simulink library "netZeroSpoolingController_ul"  (R2018b)
settings: Solver=VariableStepAuto  StartTime=0.0  StopTime=10.0  RelTol=1e-3
undefined symbols (not defined in the file or in its folder): hiLvlCtrl
libraries: simulink x2, dspsigops x1, runningAvg_ul x1
settings Model: Creator=James Reed  LastModifiedBy=mcobb

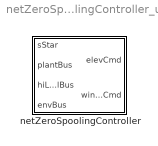
== system netZeroSpoolingController_ul ==
  netZeroSpoolingController : Subsystem  mask{L0=hiLvlCtrl.basisParams.Value(5), reelInDefl=23, reelOutDefl=0, sigmaVecInit=0}
      mask prompts: L0 "Target Tether Length"; reelInDefl "Reel In Elevator Deflection [deg]"; reelOutDefl "Reel Out Elevator Deflection [deg]"; sigmaVecInit "Init Spooling Param Vec [center width]"
      mask TypeOptions L0: TargetTetherLength/Value
      mask TypeOptions reelInDefl: ReelInElevDefl/Value
      mask TypeOptions reelOutDefl: ReelOutElevDefl/Value

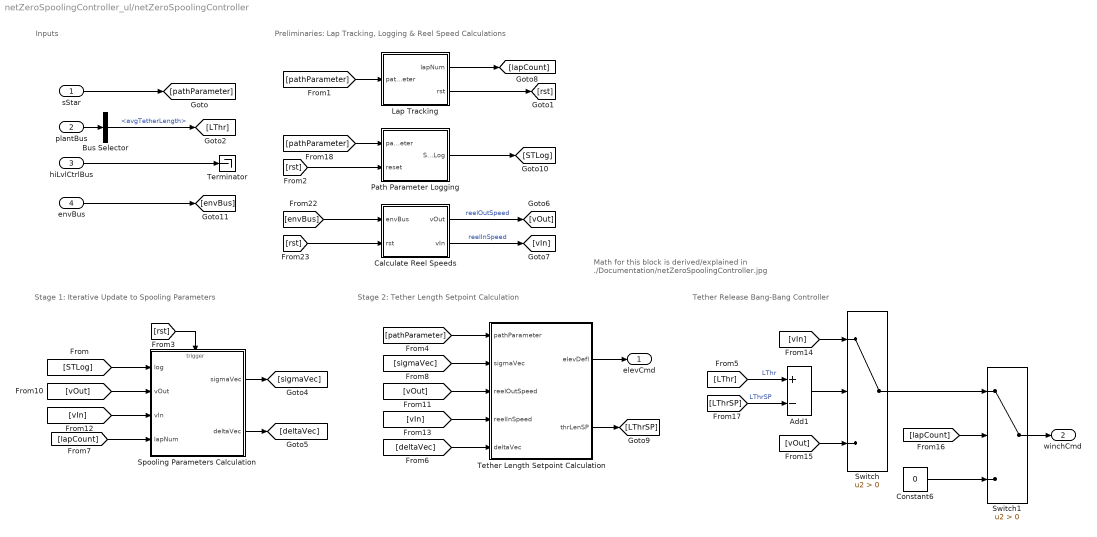
== system netZeroSpoolingController_ul/netZeroSpoolingController ==
  note: Math for this block is derived/explained in
      | ./Documentation/netZeroSpoolingController.jpg
  note: Stage 1: Iterative Update to Spooling Parameters
  note: Tether Release Bang-Bang Controller
  note: Stage 2: Tether Length Setpoint Calculation
  note: Inputs
  note: Preliminaries: Lap Tracking, Logging & Reel Speed Calculations
  "sStar " : Inport
  plantBus : Inport  Port=2  OutDataTypeStr=Bus: plantBus
  hiLvlCtrlBus : Inport  Port=3  OutDataTypeStr=Bus: hiLvlCtrlBus
  envBus : Inport  Port=4  OutDataTypeStr=Bus: envBus
  Add1 : Sum  Inputs=+-
  Bus Selector : BusSelector  OutputSignals=avgTetherLength
  Calculate Reel Speeds : Subsystem
  Constant6 : Constant  Value=0
  Lap Tracking : Subsystem
  Path Parameter Logging : Subsystem
  Spooling Parameters Calculation : Subsystem  TreatAsAtomicUnit=on
  Switch : Switch  Criteria=u2 > Threshold
  Switch1 : Switch  Criteria=u2 > Threshold
  Terminator : Terminator
  Tether Length Setpoint Calculation : Subsystem
  elevCmd : Outport
  "winchCmd " : Outport  Port=2
  wires:
  hiLvlCtrlBus/1 -> Terminator/1
  plantBus/1 -> Bus Selector/1
  "sStar "/1 -> [pathParameter]
  [rst] -> Spooling Parameters Calculation/Trigger
  Bus Selector/1 -> [LThr]  "<avgTetherLength>"
  [LThr] -> Add1/1  "LThr"
  Add1/1 -> Switch/2
  Spooling Parameters Calculation/1(sigmaVec) -> [sigmaVec]
  Spooling Parameters Calculation/2(deltaVec) -> [deltaVec]
  [vOut] -> Spooling Parameters Calculation/2(vOut)
  [vIn] -> Spooling Parameters Calculation/3(vIn)
  Switch1/1 -> "winchCmd "/1
  [LThrSP] -> Add1/2  "LThrSP"
  [vIn] -> Switch/1
  [vOut] -> Switch/3
  [lapCount] -> Switch1/2
  Switch/1 -> Switch1/1
  Constant6/1 -> Switch1/3
  [pathParameter] -> Path Parameter Logging/1(pathParameter)
  [rst] -> Path Parameter Logging/2(reset)
  Path Parameter Logging/1(SVsTLog) -> [STLog]
  [STLog] -> Spooling Parameters Calculation/1(log)
  envBus/1 -> [envBus]
  [envBus] -> Calculate Reel Speeds/1(envBus)
  Calculate Reel Speeds/1(vOut) -> [vOut]  "reelOutSpeed"
  Calculate Reel Speeds/2(vIn) -> [vIn]  "reelInSpeed"
  [rst] -> Calculate Reel Speeds/2(rst)
  [pathParameter] -> Lap Tracking/1(pathParameter)
  Lap Tracking/1(lapNum) -> [lapCount]
  Lap Tracking/2(rst) -> [rst]
  [pathParameter] -> Tether Length Setpoint Calculation/1(pathParameter)
  [sigmaVec] -> Tether Length Setpoint Calculation/2(sigmaVec)
  [vOut] -> Tether Length Setpoint Calculation/3(reelOutSpeed)
  [vIn] -> Tether Length Setpoint Calculation/4(reelInSpeed)
  [deltaVec] -> Tether Length Setpoint Calculation/5(deltaVec)
  Tether Length Setpoint Calculation/1(elevDefl) -> elevCmd/1
  Tether Length Setpoint Calculation/2(thrLenSP) -> [LThrSP]
  [lapCount] -> Spooling Parameters Calculation/4(lapNum)

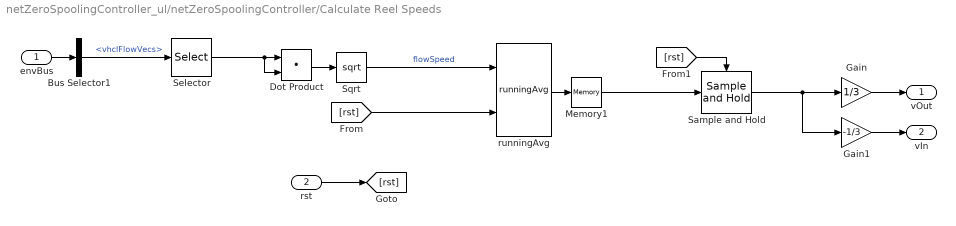
== system netZeroSpoolingController_ul/netZeroSpoolingController/Calculate Reel Speeds ==
  envBus : Inport
  rst : Inport  Port=2
  Bus Selector1 : BusSelector  OutputSignals=vhclFlowVecs
  Dot Product : DotProduct  InputSameDT=on  OutDataTypeStr=Inherit: Inherit via internal rule
  Gain : Gain  Gain=1/3
  Gain1 : Gain  Gain=-1/3
  Memory1 : Memory
  Sample and Hold : dspsigops/Sample and Hold  trig=Rising edge  initCond=0  latchinput=off
  Selector : Selector  NumberOfDimensions=2  InputPortWidth=3  IndexOptions=Select all,Index vector (dialog)  Indices=[1 3],5  OutputSizes=1,1
  Sqrt : Sqrt  SaturateOnIntegerOverflow=on
  runningAvg : runningAvg_ul/runningAvg  SystemSampleTime=-1
  vOut : Outport
  vIn : Outport  Port=2
  wires:
  Gain1/1 -> vIn/1
  Gain/1 -> vOut/1
  Sample and Hold/1 -> Gain1/1, Gain/1
  rst/1 -> [rst]
  Bus Selector1/1 -> Selector/1  "<vhclFlowVecs>"
  runningAvg/1 -> Memory1/1
  Sqrt/1 -> runningAvg/1  "flowSpeed"
  envBus/1 -> Bus Selector1/1
  Memory1/1 -> Sample and Hold/1
  [rst] -> runningAvg/2
  [rst] -> Sample and Hold/Trigger
  Selector/1 -> Dot Product/2, Dot Product/1
  Dot Product/1 -> Sqrt/1

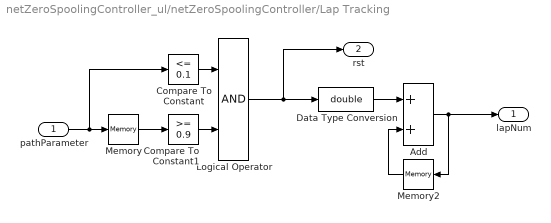
== system netZeroSpoolingController_ul/netZeroSpoolingController/Lap Tracking ==
  pathParameter : Inport
  Add : Sum
  Compare To Constant : simulink/Logic and Bit Operations/Compare To Constant  relop=<=  const=0.1  OutDataTypeStr=boolean
  Compare To Constant1 : simulink/Logic and Bit Operations/Compare To Constant  relop=>=  const=0.9  OutDataTypeStr=boolean
  Data Type Conversion : DataTypeConversion  OutDataTypeStr=double
  Logical Operator : Logic  AllPortsSameDT=off  OutDataTypeStr=boolean
  Memory : Memory
  Memory2 : Memory
  lapNum : Outport
  rst : Outport  Port=2
  wires:
  Memory/1 -> Compare To Constant1/1
  Data Type Conversion/1 -> Add/1
  Compare To Constant1/1 -> Logical Operator/2
  Add/1 -> lapNum/1, Memory2/1
  Logical Operator/1 -> rst/1, Data Type Conversion/1
  Memory2/1 -> Add/2
  pathParameter/1 -> Memory/1, Compare To Constant/1
  Compare To Constant/1 -> Logical Operator/1

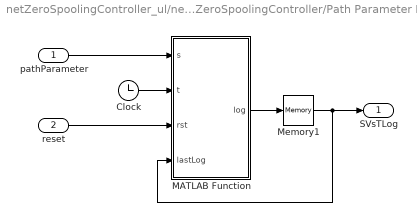
== system netZeroSpoolingController_ul/netZeroSpoolingController/Path Parameter Logging ==
  pathParameter : Inport
  reset : Inport  Port=2
  Clock : Clock
  MATLAB Function : MATLAB Function  TreatAsAtomicUnit=on
  Memory1 : Memory  InitialCondition=zeros(1000,2)
  SVsTLog : Outport
  wires:
  MATLAB Function/1(log) -> Memory1/1
  Memory1/1 -> SVsTLog/1, MATLAB Function/4(lastLog)
  reset/1 -> MATLAB Function/3(rst)
  pathParameter/1 -> MATLAB Function/1(s)
  Clock/1 -> MATLAB Function/2(t)

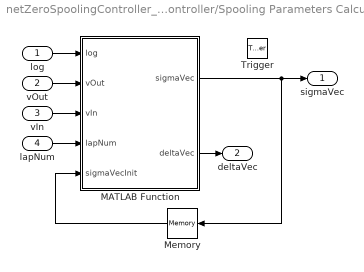
== system netZeroSpoolingController_ul/netZeroSpoolingController/Spooling Parameters Calculation ==
  log : Inport
  vOut : Inport  Port=2
  vIn : Inport  Port=3
  lapNum : Inport  Port=4
  Trigger : TriggerPort  VariantControl=Variant
  MATLAB Function : MATLAB Function  TreatAsAtomicUnit=on
  Memory : Memory  InitialCondition=sigmaVecInit  InheritSampleTime=on
  sigmaVec : Outport  InitialOutput=sigmaVecInit
  deltaVec : Outport  Port=2  InitialOutput="[0.0136    0.0097    0.0198    0.0152    0.0208]"
  wires:
  log/1 -> MATLAB Function/1(log)
  Memory/1 -> MATLAB Function/5(sigmaVecInit)
  vOut/1 -> MATLAB Function/2(vOut)
  vIn/1 -> MATLAB Function/3(vIn)
  MATLAB Function/2(deltaVec) -> deltaVec/1
  MATLAB Function/1(sigmaVec) -> Memory/1, sigmaVec/1
  lapNum/1 -> MATLAB Function/4(lapNum)

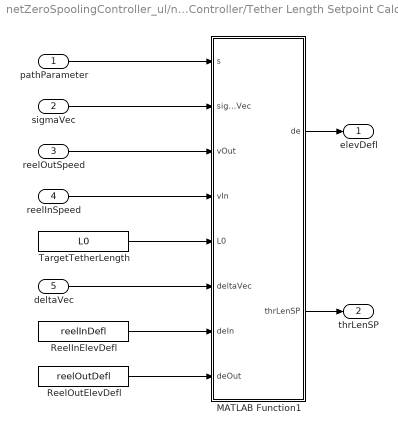
== system netZeroSpoolingController_ul/netZeroSpoolingController/Tether Length Setpoint Calculation ==
  pathParameter : Inport
  sigmaVec : Inport  Port=2
  reelOutSpeed : Inport  Port=3
  reelInSpeed : Inport  Port=4
  deltaVec : Inport  Port=5
  MATLAB Function1 : MATLAB Function  TreatAsAtomicUnit=on
  ReelInElevDefl : Constant  Value=reelInDefl
  ReelOutElevDefl : Constant  Value=reelOutDefl
  TargetTetherLength : Constant  Value=L0
  elevDefl : Outport
  thrLenSP : Outport  Port=2
  wires:
  sigmaVec/1 -> MATLAB Function1/2(sigmaVec)
  reelInSpeed/1 -> MATLAB Function1/4(vIn)
  reelOutSpeed/1 -> MATLAB Function1/3(vOut)
  pathParameter/1 -> MATLAB Function1/1(s)
  MATLAB Function1/2(thrLenSP) -> thrLenSP/1
  MATLAB Function1/1(de) -> elevDefl/1
  deltaVec/1 -> MATLAB Function1/6(deltaVec)
  ReelInElevDefl/1 -> MATLAB Function1/7(deIn)
  ReelOutElevDefl/1 -> MATLAB Function1/8(deOut)
  TargetTetherLength/1 -> MATLAB Function1/5(L0)

== matlab function netZeroSpoolingController_ul/netZeroSpoolingController/Spooling Parameters Calculation/MATLAB Function ==
  data: log input; vOut input; vIn input; lapNum input; sigmaVecInit input; sigmaVec output; deltaVec output
function [sigmaVec,deltaVec] = fcn(log,vOut,vIn,lapNum,sigmaVecInit)

sc = sigmaVecInit(1);
sw = sigmaVecInit(2);
sigmaVec = sigmaVecInit;

cleanLog = [0 0;...
    log(and(log(:,1)~=0,log(:,2)~=0),:)];
 
% Extract regions
r1 = cleanLog(and(cleanLog(:,1)>=0        ,cleanLog(:,1)<sc-sw),:);
r2 = cleanLog(and(cleanLog(:,1)>=sc-sw    ,cleanLog(:,1)<sc+sw),:);
r3 = cleanLog(and(cleanLog(:,1)>=sc+sw    ,cleanLog(:,1)<0.5+sc-sw),:);
r4 = cleanLog(and(cleanLog(:,1)>=0.5+sc-sw,cleanLog(:,1)<0.5+sc+sw),:);
r5 = cleanLog(and(cleanLog(:,1)>=0.5+sc+sw,cleanLog(:,1)<=1),:);

% Calculate average numerical derivative in each region ds/dt
ds1 = mean(diff(r1(:,1))./diff(r1(:,2)));
ds2 = mean(diff(r2(:,1))./diff(r2(:,2)));
ds3 = mean(diff(r3(:,1))./diff(r3(:,2)));
ds4 = mean(diff(r4(:,1))./diff(r4(:,2)));
ds5 = mean(diff(r5(:,1))./diff(r5(:,2)));

deltaVec = [ds1 ds2 ds3 ds4 ds5]';

dsInv = diag([1/ds1 1/ds2 1/ds3 1/ds4 1/ds5]);

V = diag([vOut vIn vOut vIn vOut]);

Delta = eye(5);
Delta(2,1) = -1;
Delta(3,2) = -1;
Delta(4,3) = -1;
Delta(5,4) = -1;

A  = [ 0  0 0.5 0.5 1]';
B1 = [ 1  1   1   1 0]';
B2 = [-1  1  -1   1 0]';

c1 = ones(1,5)*V*dsInv*Delta*(A+B1*sc);
c2 = ones(1,5)*V*dsInv*Delta*B2;
sw = min([max([-c1/c2 0]) sc]); % 0<=sw<=0.25

sigmaVec(2) = sw;

% Note: the following code alternates between updating sc and sw.
% After a bit of testing, I found that the update on sc was really screwing
% things up.  Not sure why that is at the moment, but it's kind of
% irrelevant since the update on sw alone works well enough.  Moving on.
% -MC

% Alternate updaing sc and sw each lap
% if mod(round(lapNum),2) % Odd lap number
    % Case 1, sc fixed, update sw
%     sigmaVec(1) = sc;
%     c1 = ones(1,5)*V*dsInv*Delta*(A+B1*sc);
%     c2 = ones(1,5)*V*dsInv*Delta*B2;
%     sw = min([max([-c1/c2 0]) sc]); % 0<=sw<=0.25
% else % Even lap number
%     % Case 2, sw fixed, update sc
% %     sigmaVec(2) = sw;
%     c1 = ones(1,5)*V*dsInv*Delta*(A+B2*sw);
%     c2 = ones(1,5)*V*dsInv*Delta*B1;
%     sc = min([max([-c1/c2 sw]) 0.5-sw]);
% end

% sigmaVec(1) = sc;
% sigmaVec(2) = sw;

== matlab function netZeroSpoolingController_ul/netZeroSpoolingController/Path Parameter Logging/MATLAB Function ==
  data: s input; log output; t input; rst input; lastLog input
function log = fcn(s,t,rst,lastLog)
% function that logs the path position and time into a matrix
% [pathPosition,t]
if rst
    lastLog = nan(1000,2);
end
log = lastLog;
idx = min([max([round(s*1000),1]),1000]);
log(idx,1) = s;
log(idx,2) = t;

== matlab function netZeroSpoolingController_ul/netZeroSpoolingController/Tether Length Setpoint Calculation/MATLAB Function1 ==
  data: de output; s input; thrLenSP output; sigmaVec input; vOut input; vIn input; L0 input; deltaVec input; deIn input; deOut input
function [de,thrLenSP] = fcn(s,sigmaVec,vOut,vIn,L0,deltaVec,deIn,deOut)

[de,thrLenSP] = LThrInt(s,sigmaVec,vOut,vIn,L0,deltaVec,deIn,deOut);

end
